simulink model "P7_time_sim_model"  (R2024b)
settings: Solver=VariableStepAuto  StartTime=0.0  StopTime=5  RelTol=1e-3
values from neighbouring files (symbols this model uses):
  ap = 16e-2    (= 0.16)    [P7.m]
  as = 2e-1    (= 0.2)    [P7.m]
  Da0 = 1.5e-3    (= 0.0015)    [P7.m]
  Ga = 0.112    [P7.m]
  Gf = 1/(Gs*Kd)    (= 0.25)    [P7.m]
  Gs = 0.5    [P7.m]
  R0 = 1    [P7.m]
  wp = 0.03    [P7.m]
  ws = 60    [P7.m]
libraries: cstblocks x2, simulink x2
settings Model: Creator=lucap  LastModifiedBy=lucap

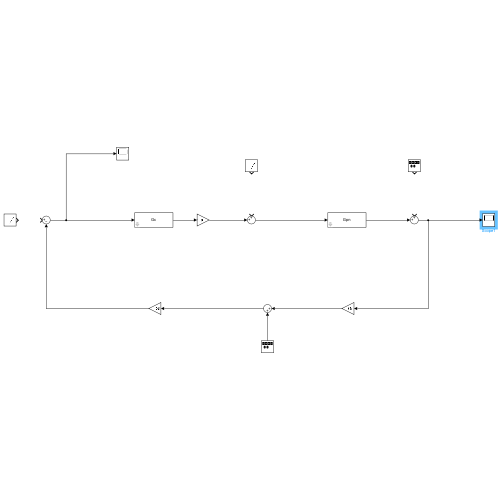
[thumbnail: Simulink's stored preview of the top-level diagram]
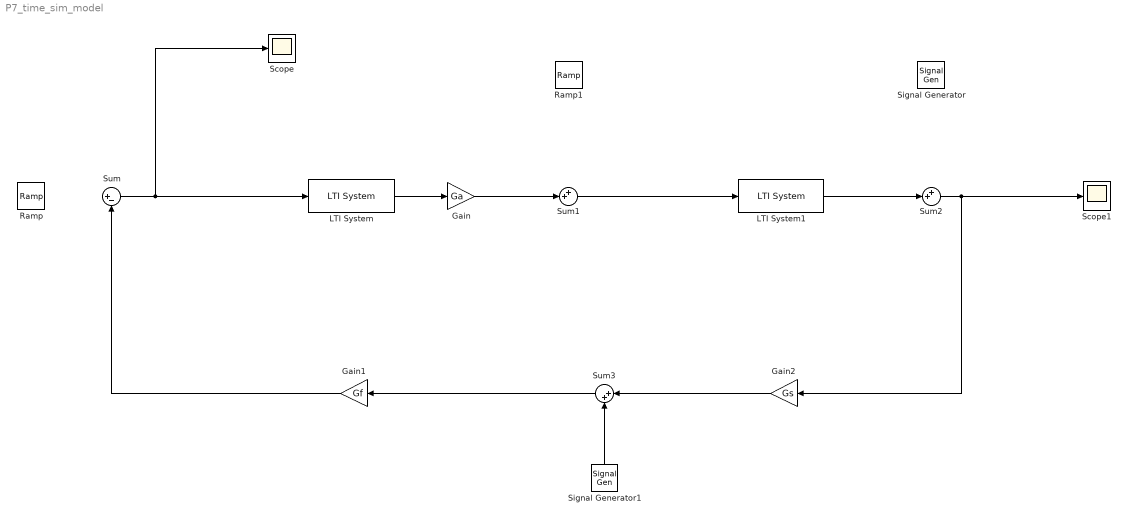
== system P7_time_sim_model ==
  Gain : Gain  Gain=Ga
  Gain1 : Gain  Gain=Gf
  Gain2 : Gain  Gain=Gs
  LTI System : cstblocks/LTI System  sys=Gc  IC=[]  PadeOrder=0
  LTI System1 : cstblocks/LTI System  sys=Gpn  IC=[]  PadeOrder=0
  Ramp : simulink/Sources/Ramp  slope=R0  start=0  InitialOutput=0
  Ramp1 : simulink/Sources/Ramp  slope=Da0  start=0  InitialOutput=0
  Scope : Scope
  Scope1 : Scope
  Signal Generator : SignalGenerator  Amplitude=ap  Frequency=wp  Units=rad/sec
  Signal Generator1 : SignalGenerator  Amplitude=as  Frequency=ws  Units=rad/sec
  Sum : Sum  Inputs=|+-
  Sum1 : Sum  Inputs=++|
  Sum2 : Sum  Inputs=++|
  Sum3 : Sum  Inputs=|++
  wires:
  Gain1/1 -> Sum/2
  Sum/1 -> Scope/1, LTI System/1
  LTI System/1 -> Gain/1
  Gain/1 -> Sum1/2
  Sum1/1 -> LTI System1/1
  LTI System1/1 -> Sum2/2
  Sum2/1 -> Scope1/1, Gain2/1
  Gain2/1 -> Sum3/1
  Sum3/1 -> Gain1/1
  Signal Generator1/1 -> Sum3/2
